simulink model "SHEV_Camaro_PwrLossMdl"  (R2018b)
settings: Solver=ode2  StartTime=0.0  StopTime=simDrv.time_s(end)  FixedStep=t_step  RelTol=1e-3
values from neighbouring files (symbols this model uses):
  A123_ESS =     [PwrLossMdl_A123Battery.mat]
  contMotTrq = [180;180;180;180;180;180;180;180;170]    [startPwrLossMdl.m]
  cs_ll = 0.15    [startPwrLossMdl.m]
  cs_ul = 0.25    [startPwrLossMdl.m]
  E85_LHV = 30000    [startPwrLossMdl.m]
  mot_gbx_rat = 4.2    [startPwrLossMdl.m]
  rho_fuel_gpL = 783    [startPwrLossMdl.m]
  simDrv = EEC_Single    [startPwrLossMdl.m]
  t_step = 0.1    [startPwrLossMdl.m]
  tire_rad_m = 0.346    [startPwrLossMdl.m]
  V_fuel_init_gal = 7    [startPwrLossMdl.m]
undefined symbols (not defined in the file or in its folder): adj_motEffMap, adjbsfc_map, adjbsfc_spdbpt, adjbsfc_trqbpt, C1, C2, DiscIntNeverNeededParam, motSpdVec, motTrqVec, N_OptResults, R0, R1, R2, soc_bpt
libraries: simulink x7, custom_func x1, dspstat3 x1
PauseFcn:
  | runOptSHEV_DP_FwdProp
settings Model: Creator=Aman-Home  LastModifiedBy=amankalia

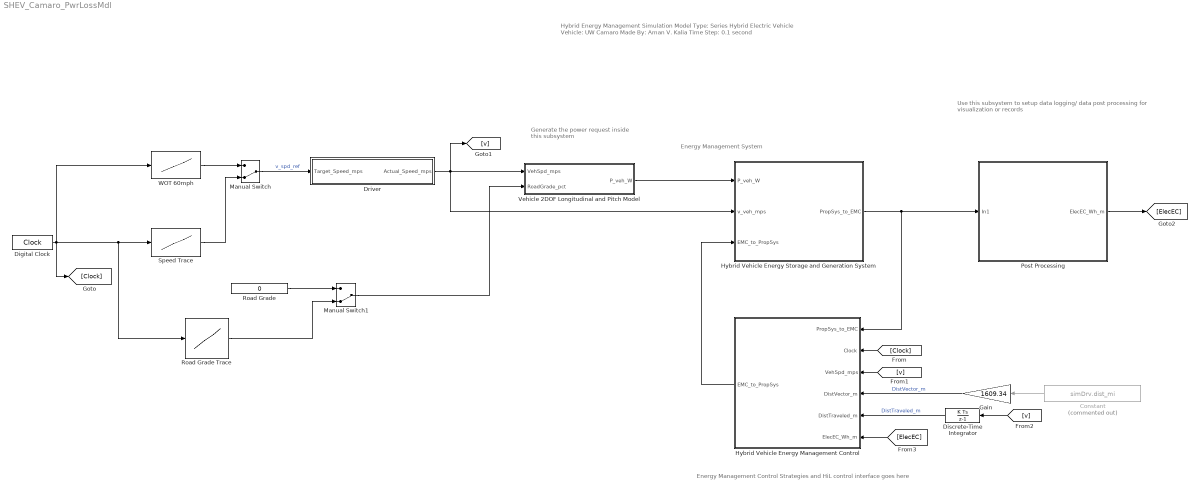
== system SHEV_Camaro_PwrLossMdl ==
  note: Energy Management Control Strategies and HiL control interface goes here
  note: Hybrid Energy Management Simulation Model
      | Type: Series Hybrid Electric Vehicle
      | Vehicle: UW Camaro
      | Made By: Aman V. Kalia
      | Time Step: 0.1 second
  note: Use this subsystem to setup data logging/ data post processing
      | for visualization or records
  note: Generate the power request inside
      | this subsystem
  note: Energy Management System
  Constant : Constant  Commented=on  Value=simDrv.dist_mi
  Digital Clock : DigitalClock  SampleTime=t_step
  Discrete-Time Integrator : DiscreteIntegrator  SampleTime=t_step  ICPrevOutput=DiscIntNeverNeededParam  ICPrevScaledInput=DiscIntNeverNeededParam
  Driver : Subsystem
  Gain : Gain  Gain=1609.34
  Hybrid Vehicle Energy Management Control : Subsystem
  Hybrid Vehicle Energy Storage and Generation System : Subsystem
  Manual Switch : ManualSwitch  CurrentSetting=0
  Manual Switch1 : ManualSwitch  CurrentSetting=0
  Post Processing : Subsystem
  Road Grade : Constant  Value=0
  Road Grade Trace : Lookup_n-D  NumberOfTableDimensions=1  BreakpointsForDimension1=simDrv.time_s  Table=simDrv.grade_pct  ExtrapMethod=Clip  InternalRulePriority=Speed  RndMeth=Simplest  InputSameDT=on
  Speed Trace : Lookup_n-D  NumberOfTableDimensions=1  BreakpointsForDimension1=simDrv.time_s  Table=simDrv.spd_mps  ExtrapMethod=Clip  InternalRulePriority=Speed  RndMeth=Simplest  InputSameDT=on
  Vehicle 2DOF Longitudinal and Pitch Model : Subsystem
  WOT 60mph : Lookup_n-D  NumberOfTableDimensions=1  BreakpointsForDimension1=[0,5,10,simDrv.time_s(end)]  Table=[0,0,60,60] * 0.447  ExtrapMethod=Clip  InternalRulePriority=Speed  RndMeth=Simplest  InputSameDT=on
  wires:
  Manual Switch/1 -> Driver/1(Target_Speed_mps)  "v_spd_ref"
  Driver/1(Actual_Speed_mps) -> [v], Hybrid Vehicle Energy Storage and Generation System/2(v_veh_mps), Vehicle 2DOF Longitudinal and Pitch Model/1(VehSpd_mps)
  Hybrid Vehicle Energy Management Control/1(EMC_to_PropSys) -> Hybrid Vehicle Energy Storage and Generation System/3(EMC_to_PropSys)
  Hybrid Vehicle Energy Storage and Generation System/1(PropSys_to_EMC) -> Hybrid Vehicle Energy Management Control/1(PropSys_to_EMC), Post Processing/1(In1)
  Vehicle 2DOF Longitudinal and Pitch Model/1(P_veh_W) -> Hybrid Vehicle Energy Storage and Generation System/1(P_veh_W)
  Manual Switch1/1 -> Vehicle 2DOF Longitudinal and Pitch Model/2(RoadGrade_pct)
  Digital Clock/1 -> WOT 60mph/1, [Clock], Road Grade Trace/1, Speed Trace/1
  Speed Trace/1 -> Manual Switch/2
  Road Grade/1 -> Manual Switch1/1
  Road Grade Trace/1 -> Manual Switch1/2
  [Clock] -> Hybrid Vehicle Energy Management Control/2(Clock)
  [v] -> Hybrid Vehicle Energy Management Control/3(VehSpd_mps)
  Constant/1 -> Gain/1
  [v] -> Discrete-Time Integrator/1
  Discrete-Time Integrator/1 -> Hybrid Vehicle Energy Management Control/5(DistTraveled_m)  "DistTraveled_m"
  Gain/1 -> Hybrid Vehicle Energy Management Control/4(DistVector_m)  "DistVector_m"
  WOT 60mph/1 -> Manual Switch/1
  Post Processing/1(ElecEC_Wh_m) -> [ElecEC]
  [ElecEC] -> Hybrid Vehicle Energy Management Control/6(ElecEC_Wh_m)

== system SHEV_Camaro_PwrLossMdl/Driver ==
  Target_Speed_mps : Inport
  Actual_Speed_mps : Outport
  wires:
  Target_Speed_mps/1 -> Actual_Speed_mps/1

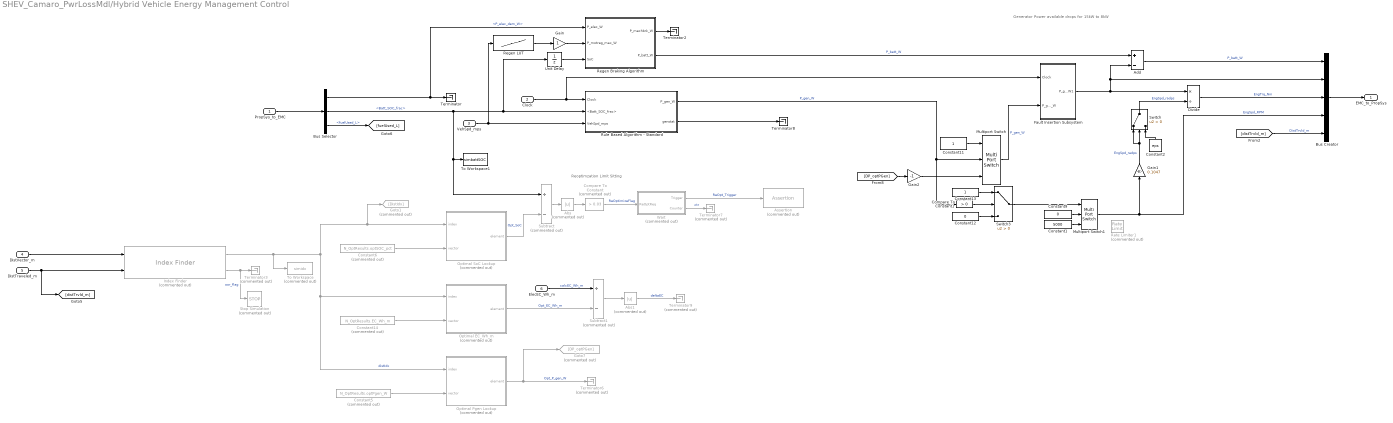
== system SHEV_Camaro_PwrLossMdl/Hybrid Vehicle Energy Management Control ==
  note: Generator Power available drops for 15kW to 8kW
  note: Reoptimzation Limit Sitting
  PropSys_to_EMC : Inport
  Clock : Inport  Port=2
  VehSpd_mps : Inport  Port=3
  DistVector_m : Inport  Port=4
  DistTraveled_m : Inport  Port=5
  ElecEC_Wh_m : Inport  Port=6
  Abs : Abs  Commented=on
  Abs1 : Abs  Commented=on
  Add : Sum  Inputs=+-
  Assertion : Assertion  Commented=on  AssertionFailFcn=set_param(bdroot,'SimulationCommand','pause');  StopWhenAssertionFail=off
  Bus Creator : BusCreator  Inputs=5
  Bus Selector : BusSelector  OutputSignals=P_elec_dem_W,Batt_SOC_frac,fuelUsed_L
  Compare To Constant : simulink/Logic and Bit Operations/Compare To Constant  Commented=on  relop=>  const=0.03  OutDataTypeStr=boolean
  Compare To Constant1 : simulink/Logic and Bit Operations/Compare To Constant  relop=>  const=0  OutDataTypeStr=boolean
  Constant1 : Constant  Value=5000
  Constant11 : Constant
  Constant12 : Constant  Value=0
  Constant13 : Constant
  Constant14 : Constant  Commented=on  Value=N_OptResults.EC_Wh_m
  Constant2 : Constant  Value=eps
  Constant5 : Constant  Commented=on  Value=N_OptResults.optPgen_W
  Constant6 : Constant  Commented=on  Value=N_OptResults.optSOC_pct
  Constant9 : Constant  Value=0
  Divide : Product  Inputs=*/
  Fault Insertion Subsystem : Subsystem  mask{FaultDec=off}
      mask prompts: FaultDec "Insert Fault"
      mask DialogControl DescGroupVar Prompt: Fault Insertion Block
      mask DialogControl DescTextVar Prompt: Select "Insert Fault" to enable fault insertion. Deselect to turn it off.
  Gain : Gain
  Gain1 : Gain  Gain=0.1047
  Gain2 : Gain  Gain=-1
  Goto1 : Goto  Commented=on  GotoTag=DistIdx
  Goto7 : Goto  Commented=on  GotoTag=DP_optPGen
  Index Finder : custom_func/Index Finder  Commented=on  SystemSampleTime=-1
  Multiport Switch : MultiPortSwitch  Inputs=2
  Multiport Switch1 : MultiPortSwitch  DataPortOrder=Zero-based contiguous  Inputs=2  zeroidx=on
  Optimal EC_Wh_m : MATLAB Function  Commented=on  TreatAsAtomicUnit=on
  Optimal Pgen Lookup : MATLAB Function  Commented=on  TreatAsAtomicUnit=on
  Optimal SoC Lookup : MATLAB Function  Commented=on  TreatAsAtomicUnit=on
  Rate Limiter1 : RateLimiter  Commented=on  RisingSlewLimit=75  FallingSlewLimit=-1000  SampleTimeMode=inherited
  Regen Braking Algorithm : Stateflow chart  TreatAsAtomicUnit=on
  Regen LUT : Lookup_n-D  NumberOfTableDimensions=1  BreakpointsForDimension1=[0 2.6 5.2 7.8 10.4 13 15.6 18.2 20.8 23.4 26 28.6 31.2 33.8 38]  Table=[0 0 -1250 -3000 -5500 -8000 -10250 -12500 -13750 -14000 -14500 -15000 -15000 -15000 -15000]  InternalRulePriority=Speed  RndMeth=Simplest  InputSameDT=on
  Rule Based Algorithm - Standard : Subsystem
  Stop Simulation : Stop  Commented=on
  Subtract : Sum  Commented=on  Inputs=+-
  Subtract1 : Sum  Commented=on  Inputs=+-
  Switch : Switch  Criteria=u2 > Threshold
  Switch3 : Switch  Criteria=u2 > Threshold
  Terminator : Terminator
  Terminator2 : Terminator
  Terminator{3,6..7,9} (4 alike) : Terminator  Commented=on
  Terminator8 : Terminator
  To Workspace : ToWorkspace  Commented=on  VariableName=simidx  SaveFormat=Timeseries  SampleTime=1
      settings: Save2DSignal=2-D array (concatenate along first dimension)
  To Workspace1 : ToWorkspace  VariableName=simbattSOC  SaveFormat=Timeseries  SampleTime=1
  Unit Delay : UnitDelay  SampleTime=-1
  Wait : Stateflow chart  Commented=on  TreatAsAtomicUnit=on
  EMC_to_PropSys : Outport
  wires:
  Bus Creator/1 -> EMC_to_PropSys/1
  Add/1 -> Bus Creator/1  "P_batt_W"
  Divide/1 -> Bus Creator/3  "EngTrq_Nm"
  Multiport Switch1/1 -> Gain1/1, Bus Creator/4  "EngSpd_RPM"
  PropSys_to_EMC/1 -> Bus Selector/1
  Bus Selector/1 -> Terminator/1, Regen Braking Algorithm/1(P_elec_W)  "<P_elec_dem_W>"
  Regen LUT/1 -> Gain/1
  Regen Braking Algorithm/1(P_mechbrk_W) -> Terminator2/1
  Gain/1 -> Regen Braking Algorithm/2(P_motreg_max_W)
  Constant9/1 -> Multiport Switch1/2
  Constant1/1 -> Multiport Switch1/3
  Switch/1 -> Divide/2  "EngSpd_radps"
  Gain1/1 -> Switch/1, Switch/2  "EngSpd_radps"
  Constant2/1 -> Switch/3
  Regen Braking Algorithm/2(P_batt_W) -> Add/1  "P_batt_W"
  Clock/1 -> Fault Insertion Subsystem/1(Clock), Rule Based Algorithm - Standard/1(Clock)
  Bus Selector/2 -> To Workspace1/1, Subtract/1, Unit Delay/1, Rule Based Algorithm - Standard/2(<Batt_SOC_frac>)  "<Batt_SOC_frac>"
  VehSpd_mps/1 -> Regen LUT/1, Rule Based Algorithm - Standard/3(VehSpd_mps)
  Switch3/1 -> Multiport Switch1/1
  DistVector_m/1 -> Index Finder/1
  DistTraveled_m/1 -> [distTrvld_m], Index Finder/2
  Index Finder/1 -> To Workspace/1, Goto1/1, Optimal SoC Lookup/1(index), Optimal EC_Wh_m/1(index), Optimal Pgen Lookup/1(index)  "distIdx"
  Index Finder/2 -> Terminator3/1, Stop Simulation/1  "oor_flag"
  Subtract/1 -> Abs/1
  Abs/1 -> Compare To Constant/1
  Compare To Constant/1 -> Wait/1(ReOptReq)  "ReOptimizeFlag"
  Wait/1(Trigger) -> Assertion/1  "ReOpt_Trigger"
  Optimal Pgen Lookup/1(element) -> Goto7/1, Terminator6/1  "Opt_P_gen_W"
  Wait/2(Counter) -> Terminator7/1  "ctr"
  Constant5/1 -> Optimal Pgen Lookup/2(vector)
  Optimal SoC Lookup/1(element) -> Subtract/2  "Opt_SoC"
  Constant6/1 -> Optimal SoC Lookup/2(vector)
  Bus Selector/3 -> [fuelUsed_L]  "<fuelUsed_L>"
  [DP_optPGen] -> Gain2/1
  Gain2/1 -> Multiport Switch/3
  Rule Based Algorithm - Standard/1(P_gen_W) -> Compare To Constant1/1, Multiport Switch/2  "P_gen_W"
  Constant11/1 -> Multiport Switch/1
  Rule Based Algorithm - Standard/2(genstat) -> Terminator8/1
  Compare To Constant1/1 -> Switch3/2
  Constant12/1 -> Switch3/3
  Constant13/1 -> Switch3/1
  [distTrvld_m] -> Bus Creator/5  "DistTrvld_m"
  Constant14/1 -> Optimal EC_Wh_m/2(vector)
  Optimal EC_Wh_m/1(element) -> Subtract1/2  "Opt_EC_Wh_m"
  ElecEC_Wh_m/1 -> Subtract1/1  "calcEC_Wh_m"
  Subtract1/1 -> Abs1/1
  Abs1/1 -> Terminator9/1  "deltaEC"
  Unit Delay/1 -> Regen Braking Algorithm/3(SoC)
  Fault Insertion Subsystem/1(P_gen_W1) -> Add/2, Bus Creator/2, Divide/1
  Multiport Switch/1 -> Fault Insertion Subsystem/2(P_gen_W)  "P_gen_W"

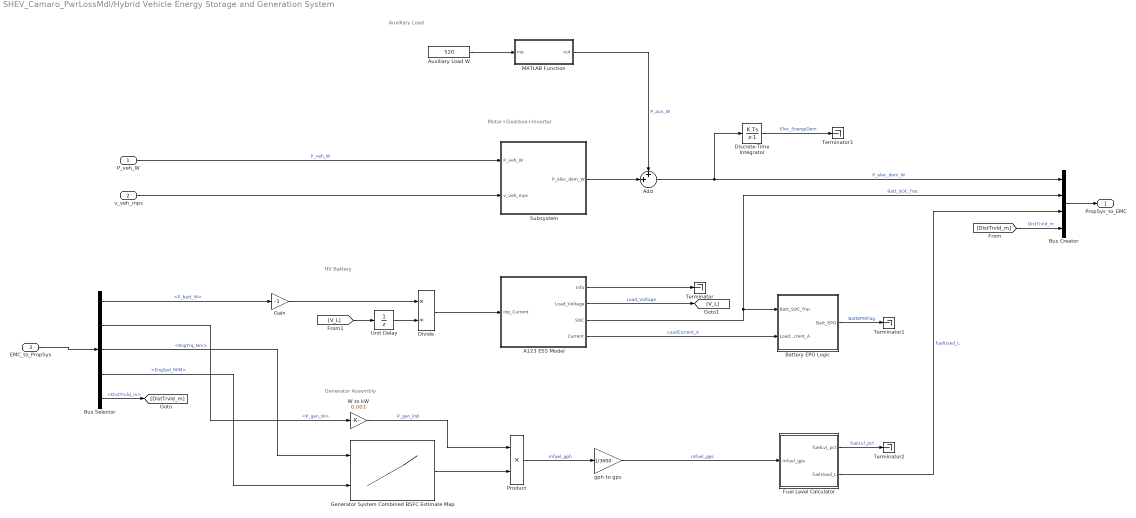
== system SHEV_Camaro_PwrLossMdl/Hybrid Vehicle Energy Storage and Generation System ==
  note: HV Battery
  note: Generator Assembly
  note: Auxiliary Load
  note: Motor+Gearbox+Inverter
  P_veh_W : Inport
  v_veh_mps : Inport  Port=2
  EMC_to_PropSys : Inport  Port=3
  A123 ESS Model : Subsystem  AncestorBlock=lib_ESS/A123 ESS Model  mask{Q_max_cell=A123_ESS.Q_cell_max_Ah, Np=A123_ESS.Np, Ns=A123_ESS.Ns, Nmod=A123_ESS.Nmod, soc_init=A123_ESS.Init_soc, soc_bpt=soc_bpt, R0=R0, R1=R1, C1=C1, R2=R2, C2=C2, t_step=t_step}
      mask prompts: Q_max_cell "Max cell capacity [Ah]:"; Np "Number of cells in parallel []:"; Ns "Numer of cells in series []:"; Nmod "Number of modules []:"; soc_init "Initial SoC/100 []:"; soc_bpt "SoC break points []:"; R0 "Internal resistance vector []:"; R1 "RC1 resistance vector []:"; C1 "RC1 capacitance vector []:"; R2 "RC2 resistance vector []:"; C2 "RC2 capacitance vector []:"; t_step "Simulation time step:"
      mask DialogControl DescGroupVar Prompt: Parameter Settings
      mask DialogControl DescTextVar Prompt: This model emulates an A123 ESS used by UW EcoCAR Team.
      mask DialogControl BatParamGroupVar Prompt: Battery Parameters
      mask DialogControl EstParamGroupVar Prompt: Estimated RC Parameters
      mask DialogControl MiscSettGroupVar Prompt: Miscellaneous Settings
  Add : Sum  Inputs=++|
  Auxiliary Load W : Constant  Value=520
  Battery EPO Logic : Subsystem
  Bus Creator : BusCreator  Inputs=4
  Bus Selector : BusSelector  OutputSignals=P_batt_W,P_gen_W,EngTrq_Nm,EngSpd_RPM,DistTrvld_m
  Discrete-Time Integrator : DiscreteIntegrator  SampleTime=t_step  ICPrevOutput=DiscIntNeverNeededParam  ICPrevScaledInput=DiscIntNeverNeededParam
  Divide : Product  Inputs=*/
  Fuel Level Calculator : Subsystem
  Gain : Gain  Gain=-1
  Generator System Combined BSFC Estimate Map : Lookup_n-D  BreakpointsForDimension1=adjbsfc_trqbpt  BreakpointsForDimension2=adjbsfc_spdbpt  Table=adjbsfc_map  InternalRulePriority=Speed  RndMeth=Simplest  InputSameDT=on
  MATLAB Function : MATLAB Function  TreatAsAtomicUnit=on
  Product : Product
  Subsystem : Subsystem
  Terminator{,1..3} (4 alike) : Terminator
  Unit Delay : UnitDelay  InitialCondition=A123_ESS.Ns * A123_ESS.Nmod * 3.4  SampleTime=-1
  W to kW : Gain  Gain=0.001
  gph to gps : Gain  Gain=1/3600
  PropSys_to_EMC : Outport
  wires:
  P_veh_W/1 -> Subsystem/1(P_veh_W)  "P_veh_W"
  v_veh_mps/1 -> Subsystem/2(v_veh_mps)
  Auxiliary Load W/1 -> MATLAB Function/1(inp)
  Subsystem/1(P_elec_dem_W) -> Add/2
  MATLAB Function/1(out) -> Add/1  "P_aux_W"
  Add/1 -> Discrete-Time Integrator/1, Bus Creator/1  "P_elec_dem_W"
  Divide/1 -> A123 ESS Model/1(Inp_Current)
  A123 ESS Model/2(Load_Voltage) -> [V_L]  "Load_Voltage"
  [V_L] -> Unit Delay/1
  A123 ESS Model/1(Info) -> Terminator/1
  A123 ESS Model/3(SOC) -> Bus Creator/2, Battery EPO Logic/1(Batt_SOC_frac)  "Batt_SOC_frac"
  Bus Selector/3 -> Generator System Combined BSFC Estimate Map/1  "<EngTrq_Nm>"
  Bus Selector/4 -> Generator System Combined BSFC Estimate Map/2  "<EngSpd_RPM>"
  EMC_to_PropSys/1 -> Bus Selector/1
  Bus Selector/1 -> Gain/1  "<P_batt_W>"
  Bus Selector/2 -> W to kW/1  "<P_gen_W>"
  Generator System Combined BSFC Estimate Map/1 -> Product/2
  W to kW/1 -> Product/1  "P_gen_kW"
  Product/1 -> gph to gps/1  "mfuel_gph"
  Bus Creator/1 -> PropSys_to_EMC/1
  Unit Delay/1 -> Divide/2
  Gain/1 -> Divide/1
  A123 ESS Model/4(Current) -> Battery EPO Logic/2(LoadCurrent_A)  "LoadCurrent_A"
  Battery EPO Logic/1(Batt_EPO) -> Terminator1/1  "BattEPOFlag"
  gph to gps/1 -> Fuel Level Calculator/1(mfuel_gps)  "mfuel_gps"
  Fuel Level Calculator/1(fuelLvl_pct) -> Terminator2/1  "fuelLvl_pct"
  Discrete-Time Integrator/1 -> Terminator3/1  "Elec_EnergyDem"
  Fuel Level Calculator/2(fuelUsed_L) -> Bus Creator/3  "fuelUsed_L"
  Bus Selector/5 -> [DistTrvld_m]  "<DistTrvld_m>"
  [DistTrvld_m] -> Bus Creator/4  "DistTrvld_m"

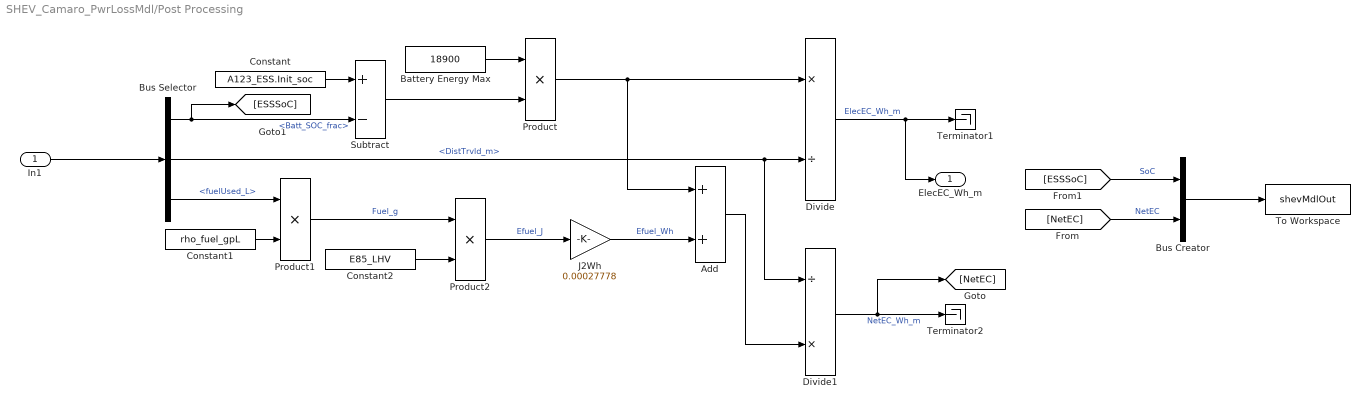
== system SHEV_Camaro_PwrLossMdl/Post Processing ==
  In1 : Inport
  Add : Sum
  Battery Energy Max : Constant  Value=18900
  Bus Creator : BusCreator  Inputs=2
  Bus Selector : BusSelector  OutputSignals=Batt_SOC_frac,DistTrvld_m,fuelUsed_L
  Constant : Constant  Value=A123_ESS.Init_soc
  Constant1 : Constant  Value=rho_fuel_gpL
  Constant2 : Constant  Value=E85_LHV
  Divide : Product  Inputs=*/
  Divide1 : Product  Inputs=/*
  J2Wh : Gain  Gain=0.00027778
  Product : Product
  Product1 : Product
  Product2 : Product
  Subtract : Sum  Inputs=+-
  Terminator1 : Terminator
  Terminator2 : Terminator
  To Workspace : ToWorkspace  VariableName=shevMdlOut  SaveFormat=Timeseries  SampleTime=-1
  ElecEC_Wh_m : Outport
  wires:
  In1/1 -> Bus Selector/1
  Bus Selector/1 -> [ESSSoC], Subtract/2  "<Batt_SOC_frac>"
  Constant/1 -> Subtract/1
  Subtract/1 -> Product/2
  Battery Energy Max/1 -> Product/1
  Product/1 -> Add/1, Divide/1
  Bus Selector/2 -> Divide1/1, Divide/2  "<DistTrvld_m>"
  Bus Selector/3 -> Product1/1  "<fuelUsed_L>"
  Divide/1 -> ElecEC_Wh_m/1, Terminator1/1  "ElecEC_Wh_m"
  Constant1/1 -> Product1/2
  Product1/1 -> Product2/1  "Fuel_g"
  Constant2/1 -> Product2/2
  Product2/1 -> J2Wh/1  "Efuel_J"
  J2Wh/1 -> Add/2  "Efuel_Wh"
  Add/1 -> Divide1/2
  Divide1/1 -> [NetEC], Terminator2/1  "NetEC_Wh_m"
  Bus Creator/1 -> To Workspace/1
  [NetEC] -> Bus Creator/2  "NetEC"
  [ESSSoC] -> Bus Creator/1  "SoC"

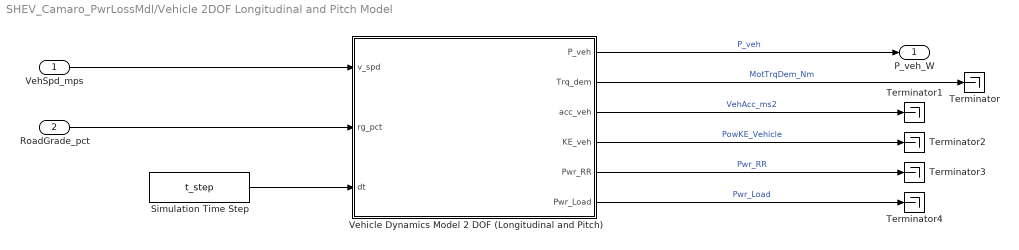
== system SHEV_Camaro_PwrLossMdl/Vehicle 2DOF Longitudinal and Pitch Model ==
  VehSpd_mps : Inport
  RoadGrade_pct : Inport  Port=2
  Simulation Time Step : Constant  Value=t_step
  Terminator{,1..4} (5 alike) : Terminator
  Vehicle Dynamics Model 2 DOF (Longitudinal and Pitch) : MATLAB Function  TreatAsAtomicUnit=on
  P_veh_W : Outport
  wires:
  VehSpd_mps/1 -> Vehicle Dynamics Model 2 DOF (Longitudinal and Pitch)/1(v_spd)
  Vehicle Dynamics Model 2 DOF (Longitudinal and Pitch)/1(P_veh) -> P_veh_W/1  "P_veh"
  RoadGrade_pct/1 -> Vehicle Dynamics Model 2 DOF (Longitudinal and Pitch)/2(rg_pct)
  Simulation Time Step/1 -> Vehicle Dynamics Model 2 DOF (Longitudinal and Pitch)/3(dt)
  Vehicle Dynamics Model 2 DOF (Longitudinal and Pitch)/2(Trq_dem) -> Terminator/1  "MotTrqDem_Nm"
  Vehicle Dynamics Model 2 DOF (Longitudinal and Pitch)/3(acc_veh) -> Terminator1/1  "VehAcc_ms2"
  Vehicle Dynamics Model 2 DOF (Longitudinal and Pitch)/4(KE_veh) -> Terminator2/1  "PowKE_Vehicle"
  Vehicle Dynamics Model 2 DOF (Longitudinal and Pitch)/5(Pwr_RR) -> Terminator3/1  "Pwr_RR"
  Vehicle Dynamics Model 2 DOF (Longitudinal and Pitch)/6(Pwr_Load) -> Terminator4/1  "Pwr_Load"

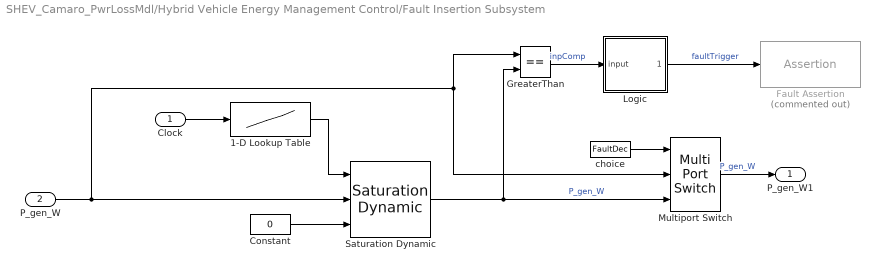
== system SHEV_Camaro_PwrLossMdl/Hybrid Vehicle Energy Management Control/Fault Insertion Subsystem ==
  Clock : Inport
  P_gen_W : Inport  Port=2
  1-D Lookup Table : Lookup_n-D  NumberOfTableDimensions=1  BreakpointsForDimension1=[0,1200,1210,simDrv.time_s(end)]  Table=[15000,15000,8000,8000]  InternalRulePriority=Speed  RndMeth=Simplest  InputSameDT=on
  Constant : Constant  Value=0
  Fault Assertion : Assertion  Commented=on  AssertionFailFcn=|  StopWhenAssertionFail=off
      | set_param(bdroot,'SimulationCommand','pause');
      | disp('## Paused due to fault insertion')
  GreaterThan : RelationalOperator  Operator===  OutDataTypeStr=boolean  RndMeth=Simplest
  Logic : Stateflow chart  TreatAsAtomicUnit=on
  Multiport Switch : MultiPortSwitch  DataPortOrder=Zero-based contiguous  Inputs=2  zeroidx=on
  Saturation Dynamic : simulink/Discontinuities/Saturation Dynamic  OutMin=[]  OutMax=[]  OutDataTypeStr=Inherit: Same as second input  OutDataType=fixdt(1, 16)  OutScaling=2^-10  DoSatur=off
  choice : Constant  Value=FaultDec
  P_gen_W1 : Outport
  wires:
  Multiport Switch/1 -> P_gen_W1/1  "P_gen_W"
  Constant/1 -> Saturation Dynamic/3
  Clock/1 -> 1-D Lookup Table/1
  P_gen_W/1 -> Multiport Switch/2, GreaterThan/1, Saturation Dynamic/2
  1-D Lookup Table/1 -> Saturation Dynamic/1
  Saturation Dynamic/1 -> GreaterThan/2, Multiport Switch/3  "P_gen_W"
  choice/1 -> Multiport Switch/1
  GreaterThan/1 -> Logic/1(input)  "inpComp"
  Logic/1(trigger) -> Fault Assertion/1  "faultTrigger"

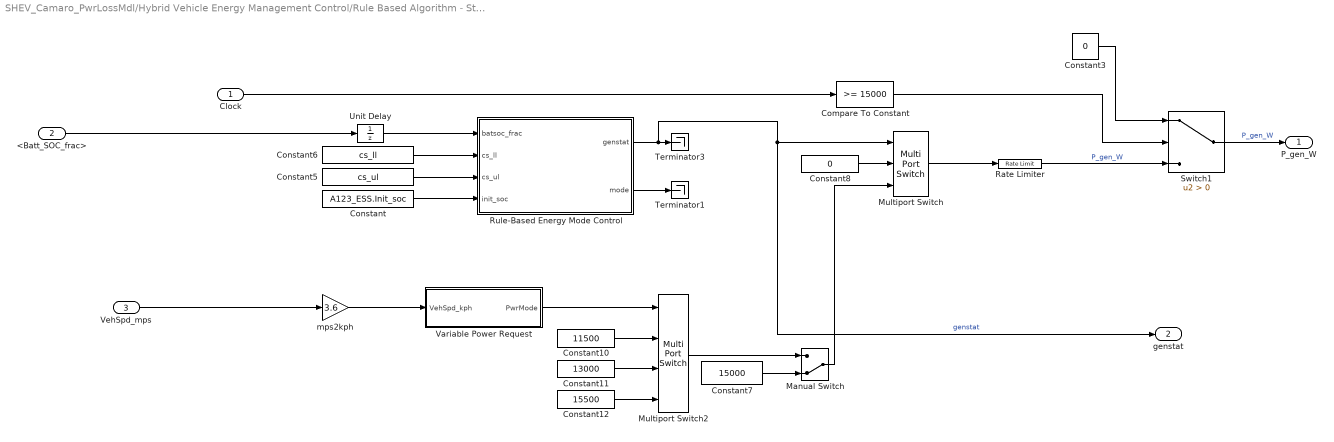
== system SHEV_Camaro_PwrLossMdl/Hybrid Vehicle Energy Management Control/Rule Based Algorithm - Standard ==
  Clock : Inport
  <Batt_SOC_frac> : Inport  Port=2
  VehSpd_mps : Inport  Port=3
  Compare To Constant : simulink/Logic and Bit Operations/Compare To Constant  relop=>=  const=15000  OutDataTypeStr=boolean
  Constant : Constant  Value=A123_ESS.Init_soc
  Constant10 : Constant  Value=11500
  Constant11 : Constant  Value=13000
  Constant12 : Constant  Value=15500
  Constant3 : Constant  Value=0
  Constant5 : Constant  Value=cs_ul
  Constant6 : Constant  Value=cs_ll
  Constant7 : Constant  Value=15000
  Constant8 : Constant  Value=0
  Manual Switch : ManualSwitch  CurrentSetting=0
  Multiport Switch : MultiPortSwitch  DataPortOrder=Zero-based contiguous  Inputs=2  zeroidx=on
  Multiport Switch2 : MultiPortSwitch  DataPortOrder=Zero-based contiguous  zeroidx=on
  Rate Limiter : RateLimiter  RisingSlewLimit=250  FallingSlewLimit=-4500  SampleTimeMode=inherited
  Rule-Based Energy Mode Control : Stateflow chart  TreatAsAtomicUnit=on
  Switch1 : Switch  Criteria=u2 > Threshold
  Terminator1 : Terminator
  Terminator3 : Terminator
  Unit Delay : UnitDelay  SampleTime=-1
  Variable Power Request : MATLAB Function  TreatAsAtomicUnit=on
  mps2kph : Gain  Gain=3.6
  P_gen_W : Outport
  genstat : Outport  Port=2
  wires:
  Multiport Switch2/1 -> Manual Switch/1
  Constant12/1 -> Multiport Switch2/4
  Constant11/1 -> Multiport Switch2/3
  Variable Power Request/1(PwrMode) -> Multiport Switch2/1
  Constant3/1 -> Switch1/1
  <Batt_SOC_frac>/1 -> Unit Delay/1
  Constant/1 -> Rule-Based Energy Mode Control/4(init_soc)
  Constant10/1 -> Multiport Switch2/2
  Constant8/1 -> Multiport Switch/2
  Clock/1 -> Compare To Constant/1
  Multiport Switch/1 -> Rate Limiter/1
  Rule-Based Energy Mode Control/2(mode) -> Terminator1/1
  Constant7/1 -> Manual Switch/2
  Rule-Based Energy Mode Control/1(genstat) -> genstat/1, Multiport Switch/1, Terminator3/1  "genstat"
  VehSpd_mps/1 -> mps2kph/1
  Unit Delay/1 -> Rule-Based Energy Mode Control/1(batsoc_frac)
  mps2kph/1 -> Variable Power Request/1(VehSpd_kph)
  Constant5/1 -> Rule-Based Energy Mode Control/3(cs_ul)
  Compare To Constant/1 -> Switch1/2
  Rate Limiter/1 -> Switch1/3  "P_gen_W"
  Constant6/1 -> Rule-Based Energy Mode Control/2(cs_ll)
  Manual Switch/1 -> Multiport Switch/3
  Switch1/1 -> P_gen_W/1  "P_gen_W"

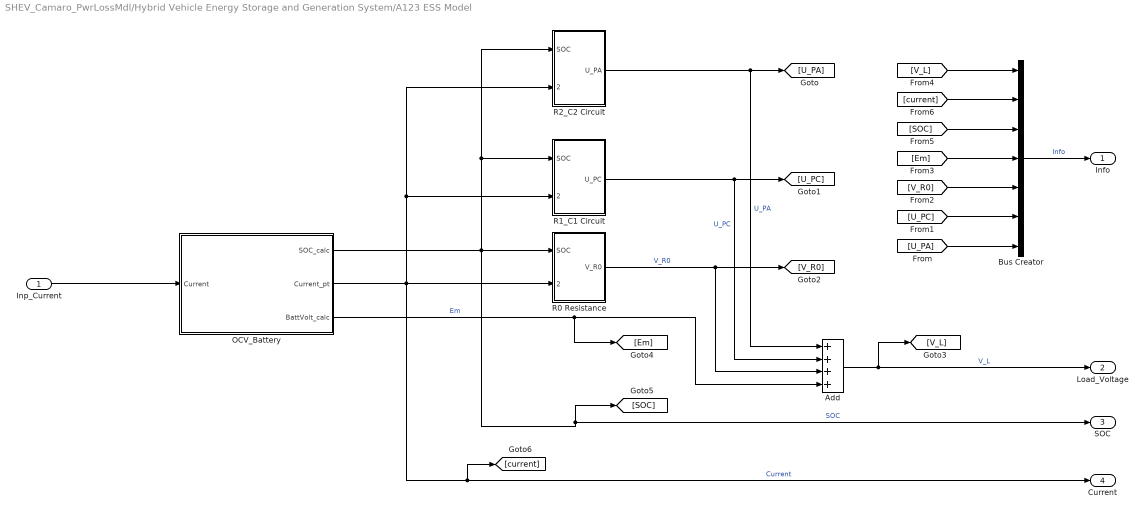
== system SHEV_Camaro_PwrLossMdl/Hybrid Vehicle Energy Storage and Generation System/A123 ESS Model ==
  Inp_Current : Inport
  Add : Sum  Inputs=++++
  Bus Creator : BusCreator  Inputs=7
  OCV_Battery : Subsystem
  R0 Resistance : Subsystem
  R1_C1 Circuit : Subsystem
  R2_C2 Circuit : Subsystem
  Info : Outport
  Load_Voltage : Outport  Port=2
  SOC : Outport  Port=3
  Current : Outport  Port=4
  wires:
  [SOC] -> Bus Creator/3
  [U_PA] -> Bus Creator/7
  Inp_Current/1 -> OCV_Battery/1(Current)
  [current] -> Bus Creator/2
  Add/1 -> Load_Voltage/1, [V_L]  "V_L"
  [Em] -> Bus Creator/4
  R0 Resistance/1(V_R0) -> [V_R0], Add/3  "V_R0"
  R2_C2 Circuit/1(U_PA) -> Add/1, [U_PA]  "U_PA"
  OCV_Battery/2(Current_pt) -> Current/1, [current], R2_C2 Circuit/2(Current), R1_C1 Circuit/2(Current), R0 Resistance/2(Current)  "Current"
  OCV_Battery/1(SOC_calc) -> SOC/1, [SOC], R2_C2 Circuit/1(SOC), R1_C1 Circuit/1(SOC), R0 Resistance/1(SOC)  "SOC"
  R1_C1 Circuit/1(U_PC) -> Add/2, [U_PC]  "U_PC"
  [U_PC] -> Bus Creator/6
  OCV_Battery/3(BattVolt_calc) -> [Em], Add/4  "Em"
  [V_R0] -> Bus Creator/5
  Bus Creator/1 -> Info/1  "Info"
  [V_L] -> Bus Creator/1

== system SHEV_Camaro_PwrLossMdl/Hybrid Vehicle Energy Storage and Generation System/Battery EPO Logic ==
  note: Discharge Current is negative
  Batt_SOC_frac : Inport
  LoadCurrent_A : Inport  Port=2
  10-second average : dspstat3/Moving Average  Method=Sliding window  ForgettingFactorPort=off  SpecifyWindowLength=on  WindowLength=1000  ForgettingFactor=0.9  SimulateUsing=Code generation
  10sec Discharge Limit Table A123 : Lookup_n-D  BreakpointsForDimension1=A123_ESS.cellTempbpt_C  BreakpointsForDimension2=A123_ESS.socbpt  Table=A123_ESS.DchgCurrLim_10sAvg_A  InternalRulePriority=Speed  RndMeth=Simplest  InputSameDT=on
  Battery EPO Constraint Logic : Stateflow chart  TreatAsAtomicUnit=on
  CellTemp degC : Constant  Value=35
  Gain1 : Gain  Gain=-1
  Batt_EPO : Outport
  wires:
  Batt_SOC_frac/1 -> 10sec Discharge Limit Table A123/2
  LoadCurrent_A/1 -> 10-second average/1
  Battery EPO Constraint Logic/1(epo_flag) -> Batt_EPO/1  "Batt_EPO"
  10-second average/1 -> Battery EPO Constraint Logic/2(LoadCurr)  "LoadCurrent_10sAvg_A"
  CellTemp degC/1 -> 10sec Discharge Limit Table A123/1
  Gain1/1 -> Battery EPO Constraint Logic/1(DchgCurrLim)
  10sec Discharge Limit Table A123/1 -> Gain1/1

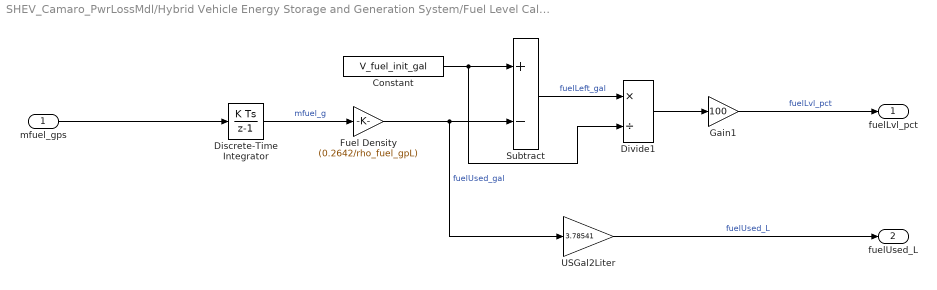
== system SHEV_Camaro_PwrLossMdl/Hybrid Vehicle Energy Storage and Generation System/Fuel Level Calculator ==
  mfuel_gps : Inport
  Constant : Constant  Value=V_fuel_init_gal
  Discrete-Time Integrator : DiscreteIntegrator  SampleTime=-1  ICPrevOutput=DiscIntNeverNeededParam  ICPrevScaledInput=DiscIntNeverNeededParam
  Divide1 : Product  Inputs=*/
  Fuel Density : Gain  Gain=(0.2642/rho_fuel_gpL)
  Gain1 : Gain  Gain=100
  Subtract : Sum  Inputs=+-
  USGal2Liter : Gain  Gain=3.78541
  fuelLvl_pct : Outport
  fuelUsed_L : Outport  Port=2
  wires:
  Divide1/1 -> Gain1/1
  Subtract/1 -> Divide1/1  "fuelLeft_gal"
  Fuel Density/1 -> USGal2Liter/1, Subtract/2  "fuelUsed_gal"
  Constant/1 -> Divide1/2, Subtract/1
  Discrete-Time Integrator/1 -> Fuel Density/1  "mfuel_g"
  mfuel_gps/1 -> Discrete-Time Integrator/1
  Gain1/1 -> fuelLvl_pct/1  "fuelLvl_pct"
  USGal2Liter/1 -> fuelUsed_L/1  "fuelUsed_L"

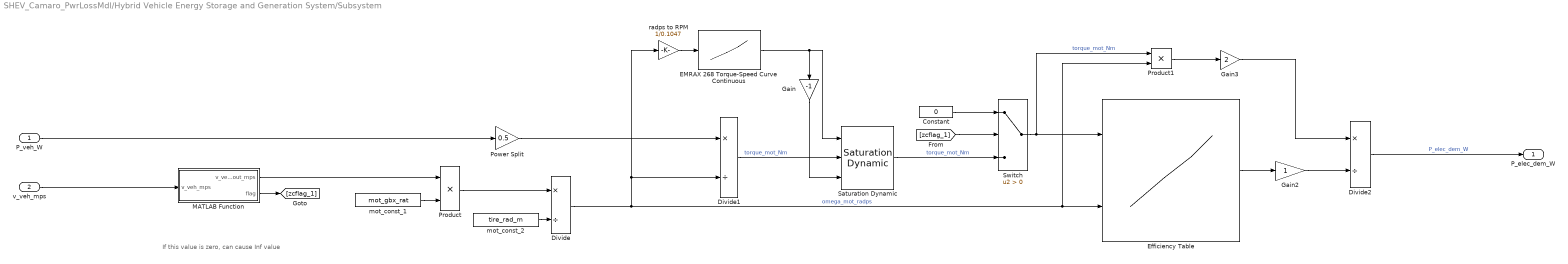
== system SHEV_Camaro_PwrLossMdl/Hybrid Vehicle Energy Storage and Generation System/Subsystem ==
  note: If this value is zero, can cause Inf value
  P_veh_W : Inport
  v_veh_mps : Inport  Port=2
  Constant : Constant  Value=0
  Divide : Product  Inputs=*/
  Divide1 : Product  Inputs=*/
  Divide2 : Product  Inputs=*/
  EMRAX 268 Torque-Speed Curve Continuous : Lookup_n-D  NumberOfTableDimensions=1  BreakpointsForDimension1=motSpdVec  Table=contMotTrq  InternalRulePriority=Speed  RndMeth=Simplest  InputSameDT=on
  Efficiency Table : Lookup_n-D  BreakpointsForDimension1=motTrqVec  BreakpointsForDimension2=motSpdVec  Table=adj_motEffMap  ExtrapMethod=Clip  UseLastTableValue=on  InternalRulePriority=Speed  RndMeth=Simplest  InputSameDT=on
  Gain : Gain  Gain=-1
  Gain2 : Gain
  Gain3 : Gain  Gain=2
  MATLAB Function : MATLAB Function  TreatAsAtomicUnit=on
  Power Split : Gain  Gain=0.5
  Product : Product
  Product1 : Product
  Saturation Dynamic : simulink/Discontinuities/Saturation Dynamic  OutMin=[]  OutMax=[]  OutDataTypeStr=Inherit: Same as second input  OutDataType=fixdt(1, 16)  OutScaling=2^-10  DoSatur=off
  Switch : Switch  Criteria=u2 > Threshold
  mot_const_1 : Constant  Value=mot_gbx_rat
  mot_const_2 : Constant  Value=tire_rad_m
  radps to RPM : Gain  Gain=1/0.1047
  P_elec_dem_W : Outport
  wires:
  Saturation Dynamic/1 -> Switch/3  "torque_mot_Nm"
  [zcflag_1] -> Switch/2
  Switch/1 -> Product1/1, Efficiency Table/1  "torque_mot_Nm"
  Product/1 -> Divide/1
  radps to RPM/1 -> EMRAX 268 Torque-Speed Curve Continuous/1
  Constant/1 -> Switch/1
  MATLAB Function/1(v_veh_out_mps) -> Product/1
  Gain/1 -> Saturation Dynamic/3
  mot_const_1/1 -> Product/2
  EMRAX 268 Torque-Speed Curve Continuous/1 -> Gain/1, Saturation Dynamic/1
  Power Split/1 -> Divide1/1
  v_veh_mps/1 -> MATLAB Function/1(v_veh_mps)
  P_veh_W/1 -> Power Split/1
  Efficiency Table/1 -> Gain2/1
  Divide1/1 -> Saturation Dynamic/2  "torque_mot_Nm"
  mot_const_2/1 -> Divide/2
  Divide/1 -> Divide1/2, radps to RPM/1, Product1/2, Efficiency Table/2  "omega_mot_radps"
  MATLAB Function/2(flag) -> [zcflag_1]
  Product1/1 -> Gain3/1
  Divide2/1 -> P_elec_dem_W/1  "P_elec_dem_W"
  Gain2/1 -> Divide2/2
  Gain3/1 -> Divide2/1

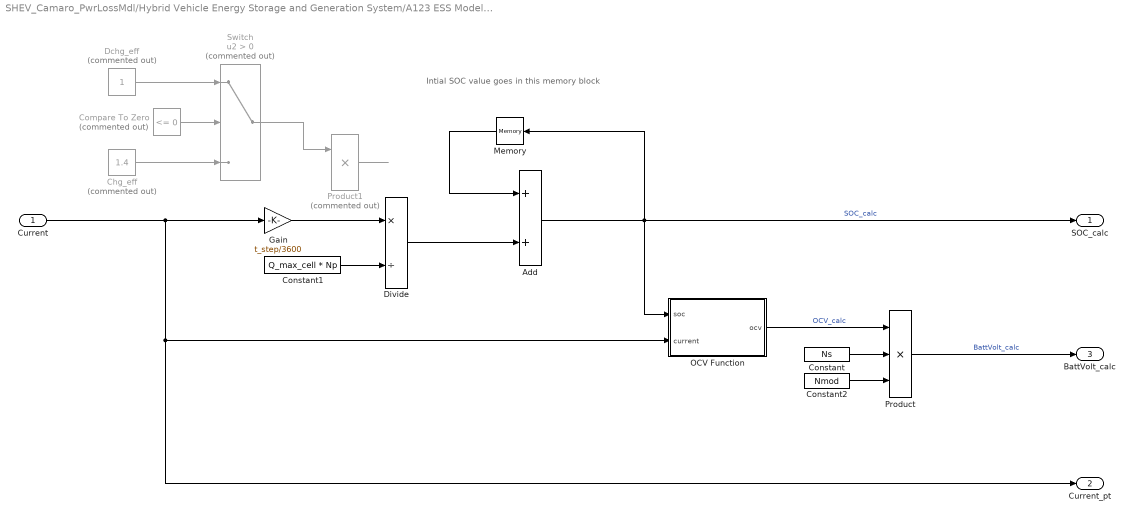
== system SHEV_Camaro_PwrLossMdl/Hybrid Vehicle Energy Storage and Generation System/A123 ESS Model/OCV_Battery ==
  note: Intial SOC value goes in this memory block
  Current : Inport
  Add : Sum
  Chg_eff : Constant  Commented=on  Value=1.4
  Compare To Zero : simulink/Logic and Bit Operations/Compare To Zero  Commented=on  relop=<=  OutDataTypeStr=boolean
  Constant : Constant  Value=Ns
  Constant1 : Constant  Value=Q_max_cell * Np
  Constant2 : Constant  Value=Nmod
  Dchg_eff : Constant  Commented=on
  Divide : Product  Inputs=*/
  Gain : Gain  Gain=t_step/3600
  Memory : Memory  InitialCondition=soc_init  InheritSampleTime=on  LinearizeAsDelay=on
  OCV Function : MATLAB Function  TreatAsAtomicUnit=on
  Product : Product  Inputs=3
  Product1 : Product  Commented=on
  Switch : Switch  Commented=on  Criteria=u2 > Threshold
  SOC_calc : Outport
  Current_pt : Outport  Port=2
  BattVolt_calc : Outport  Port=3
  wires:
  Current/1 -> OCV Function/2(current), Current_pt/1, Gain/1
  Gain/1 -> Divide/1
  Memory/1 -> Add/1
  Constant2/1 -> Product/3
  OCV Function/1(ocv) -> Product/1  "OCV_calc"
  Constant1/1 -> Divide/2
  Add/1 -> SOC_calc/1, OCV Function/1(soc), Memory/1  "SOC_calc"
  Constant/1 -> Product/2
  Divide/1 -> Add/2
  Product/1 -> BattVolt_calc/1  "BattVolt_calc"
  Compare To Zero/1 -> Switch/2
  Dchg_eff/1 -> Switch/1
  Chg_eff/1 -> Switch/3
  Switch/1 -> Product1/1
  Product1/1 -> ?

== system SHEV_Camaro_PwrLossMdl/Hybrid Vehicle Energy Storage and Generation System/A123 ESS Model/R0 Resistance ==
  SOC : Inport
  Current : Inport  Port=2
  Compare To Zero : simulink/Logic and Bit Operations/Compare To Zero  relop=>  OutDataTypeStr=boolean
  Product : Product
  R0 LUT Chg : Lookup_n-D  NumberOfTableDimensions=1  BreakpointsForDimension1=soc_bpt  Table=R0 * 0.05  InternalRulePriority=Speed  RndMeth=Simplest  InputSameDT=on
  R0 LUT Dchg : Lookup_n-D  NumberOfTableDimensions=1  BreakpointsForDimension1=soc_bpt  Table=R0*0.25  InternalRulePriority=Speed  RndMeth=Simplest  InputSameDT=on
  Switch : Switch  Criteria=u2 > Threshold
  V_R0 : Outport
  wires:
  R0 LUT Chg/1 -> Switch/1  "R0"
  SOC/1 -> R0 LUT Chg/1, R0 LUT Dchg/1
  Current/1 -> Compare To Zero/1, Product/2
  Product/1 -> V_R0/1
  Switch/1 -> Product/1
  Compare To Zero/1 -> Switch/2
  R0 LUT Dchg/1 -> Switch/3  "R0"

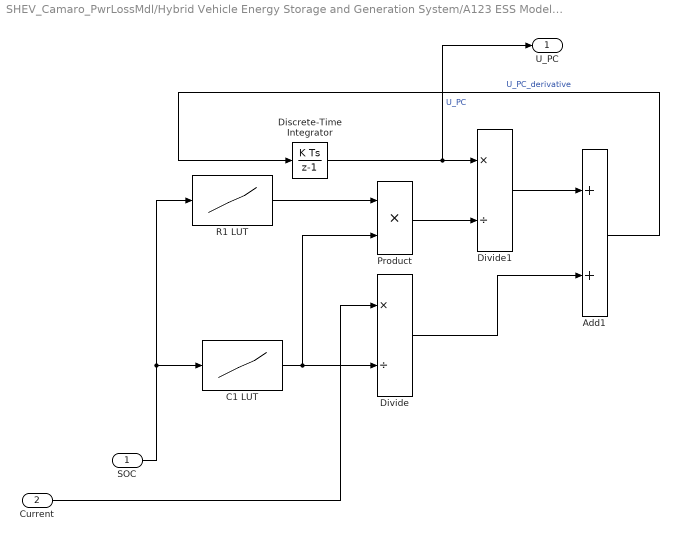
== system SHEV_Camaro_PwrLossMdl/Hybrid Vehicle Energy Storage and Generation System/A123 ESS Model/R1_C1 Circuit ==
  SOC : Inport
  Current : Inport  Port=2
  Add1 : Sum
  C1 LUT : Lookup_n-D  NumberOfTableDimensions=1  BreakpointsForDimension1=soc_bpt  Table=C1  InternalRulePriority=Speed  RndMeth=Simplest  InputSameDT=on
  Discrete-Time Integrator : DiscreteIntegrator  SampleTime=-1  ICPrevOutput=DiscIntNeverNeededParam  ICPrevScaledInput=DiscIntNeverNeededParam
  Divide : Product  Inputs=*/
  Divide1 : Product  Inputs=*/
  Product : Product
  R1 LUT : Lookup_n-D  NumberOfTableDimensions=1  BreakpointsForDimension1=soc_bpt  Table=R1  InternalRulePriority=Speed  RndMeth=Simplest  InputSameDT=on
  U_PC : Outport
  wires:
  Product/1 -> Divide1/2
  SOC/1 -> R1 LUT/1, C1 LUT/1
  Divide1/1 -> Add1/1
  C1 LUT/1 -> Product/2, Divide/2
  Divide/1 -> Add1/2
  R1 LUT/1 -> Product/1
  Discrete-Time Integrator/1 -> U_PC/1, Divide1/1  "U_PC"
  Add1/1 -> Discrete-Time Integrator/1  "U_PC_derivative"
  Current/1 -> Divide/1

== system SHEV_Camaro_PwrLossMdl/Hybrid Vehicle Energy Storage and Generation System/A123 ESS Model/R2_C2 Circuit ==
  SOC : Inport
  Current : Inport  Port=2
  Add1 : Sum
  C2 LUT : Lookup_n-D  NumberOfTableDimensions=1  BreakpointsForDimension1=soc_bpt  Table=C2  InternalRulePriority=Speed  RndMeth=Simplest  InputSameDT=on
  Discrete-Time Integrator : DiscreteIntegrator  SampleTime=-1  ICPrevOutput=DiscIntNeverNeededParam  ICPrevScaledInput=DiscIntNeverNeededParam
  Divide : Product  Inputs=*/
  Divide1 : Product  Inputs=*/
  Product : Product
  R2 LUT : Lookup_n-D  NumberOfTableDimensions=1  BreakpointsForDimension1=soc_bpt  Table=R2  InternalRulePriority=Speed  RndMeth=Simplest  InputSameDT=on
  U_PA : Outport
  wires:
  Product/1 -> Divide1/2
  SOC/1 -> R2 LUT/1, C2 LUT/1
  Divide1/1 -> Add1/1
  C2 LUT/1 -> Product/2, Divide/2
  Divide/1 -> Add1/2
  R2 LUT/1 -> Product/1
  Discrete-Time Integrator/1 -> U_PA/1, Divide1/1  "U_PA"
  Add1/1 -> Discrete-Time Integrator/1  "U_PA_derivative"
  Current/1 -> Divide/1

== matlab function SHEV_Camaro_PwrLossMdl/Hybrid Vehicle Energy Storage and Generation System/Subsystem/MATLAB Function ==
  data: v_veh_mps input; v_veh_out_mps output; flag output
function [v_veh_out_mps,flag] = zerocheck(v_veh_mps)
    % Checks if the input speed is zero. 
    % If zero: sets the flag = 1, to change torque value to zero.
    % If not zero: sets the flag = 0, no change to the the torque value.
    
    if v_veh_mps == 0
        flag = 1;
        v_veh_out_mps = v_veh_mps;
    else
        flag = 0;
        v_veh_out_mps = v_veh_mps;
    end
end

== matlab function SHEV_Camaro_PwrLossMdl/Hybrid Vehicle Energy Storage and Generation System/MATLAB Function ==
  data: inp input; out output
function out = addnoise(inp)
snr = 25;

out = awgn(inp,snr,'measured');

== matlab function SHEV_Camaro_PwrLossMdl/Vehicle 2DOF Longitudinal and Pitch Model/Vehicle Dynamics Model 2 DOF (Longitudinal and Pitch) ==
  data: v_spd input; P_veh output; rg_pct input; dt input; Trq_dem output; acc_veh output; KE_veh output; Pwr_RR output; Pwr_Load output
function [P_veh, Trq_dem, acc_veh, KE_veh, Pwr_RR, Pwr_Load] = vehdyn2dof(v_spd,rg_pct,dt)
    % DESCRIPTION: The 2DOF Longitudinal and Pitch Model for the vehicle
    % uses the longitudinal road load equation comprising of Aerodynamic
    % Resistance, Climbing Resistance, Rolling Resistance as resistive
    % forces on the vehicle.
    %
    % F_veh [N] = F_trac + F_ar + F_cr + F_rr;  --------- (1)
    % P_veh [W] = F_veh [N] * v_veh [m/s];      --------- (2)
    %
    % Note: Pitch dynamics will be added to the model once COG height for
    % the car is determined. Currently only 1DOF longitudinal dynamics
    % exist.
    
    %% Pre-processing
    persistent v_spd_old
    if isempty(v_spd_old)
        v_spd_old = v_spd;
        flag = 1;
    else
        flag = 0;
    end
    alpha = atan(rg_pct/100);
    
    %% Static Parameters
    % -- Vehicle
    A_veh = 0.4;        % [m^2]
    C_d = 0.34;         % drag coefficient [-]
    m_veh = 2012;       %1875;       % [kg]
    P_tire = 32;        % [psi]
    R_tire = 0.346;     % [m]
    N_drvnWhl = 2;      % [-]
    Rat_gbx = 4.2;
    
    % -- Environment
    g = 9.81;           % acceleration due to gravity [m/s^2]
    rho_air = 1.225;    % STP density [kg/m^3]
    
    %% Dynamic Parameters
    C_rr = 0.005 + ((0.06895/P_tire) * ...
        (0.01 + (0.0095 * ((2.778 * (10^-3) * v_spd)^2))));            
    % function of tire pressure and vehicle speed [psi, mps]
    
    %% Vehicle Power Calculation
    if flag == 1
        P_veh = 0;
        Trq_dem = 0; 
        acc_veh = 0;
        KE_veh = 0;
        Pwr_RR = 0;
        Pwr_Load = 0;
    else
        acc_veh = (v_spd - v_spd_old)/dt;
        P_veh = ((m_veh * acc_veh) + ...
            (0.5 * rho_air * A_veh * C_d * (v_spd ^ 2)) + ...
            (m_veh * g * sin(alpha)) + ...
            (C_rr * m_veh * g)) * (v_spd);
        Trq_dem = ((P_veh/v_spd) * R_tire)/((N_drvnWhl * Rat_gbx));
        KE_veh = 0.5 * m_veh * ((v_spd^2) - (v_spd_old^2));
        v_spd_old = v_spd;
        Pwr_RR = (C_rr * m_veh * g) * (v_spd);
        Pwr_Load = ((0.5 * rho_air * A_veh * C_d * (v_spd ^ 2)) + ...
            (m_veh * g * sin(alpha)) + ...
            (C_rr * m_veh * g)) * (v_spd);
    end
    
end

== stateflow chart SHEV_Camaro_PwrLossMdl/Hybrid Vehicle Energy Management Control/Regen Braking Algorithm ==
  note: %P_reg_W
  state NoBraking
    du:
    P_reg_W = 0;
    P_mechbrk_W = 0;
    P_batt_W = P_elec_W;
  state Braking
    state RegenDisabled
      du:
      P_reg_W = 0;
      P_mechbrk_W = P_elec_W;
      P_batt_W = 0;
    state RegenEnabled
      state LightBraking
        du:
        P_reg_W = P_elec_W;
        P_mechbrk_W = P_elec_W - P_reg_W;
        P_batt_W = P_reg_W;
      state HeavyBraking
        du:
        P_reg_W = P_motreg_max_W;
        P_mechbrk_W = P_elec_W - P_reg_W;
        P_batt_W = P_reg_W;
      (default) -> LightBraking
      LightBraking -> HeavyBraking : [P_elec_W <= ...
          | P_motreg_max_W]
      HeavyBraking -> LightBraking : [P_elec_W >= ...
          | P_motreg_max_W]
    (default) -> RegenDisabled
    RegenDisabled -> RegenEnabled : [SoC <= 0.95]
    RegenEnabled -> RegenDisabled : [SoC > 0.95]
  (default) -> NoBraking
  NoBraking -> Braking : [P_elec_W < 0]
  Braking -> NoBraking : [P_elec_W >= 0]
  data: P_elec_W input; P_motreg_max_W input; P_mechbrk_W output double; P_batt_W output double; P_reg_W local double; SoC input

== stateflow chart SHEV_Camaro_PwrLossMdl/Hybrid Vehicle Energy Storage and Generation System/Battery EPO Logic/Battery EPO Constraint Logic ==
  state NoEPO
    du:
    epo_flag = 0;
  state EPO
    du:
    epo_flag = 1;
  (default) -> NoEPO
  NoEPO -> EPO : [LoadCurr < DchgCurrLim]
  EPO -> NoEPO : [LoadCurr >= DchgCurrLim]
  data: DchgCurrLim input; LoadCurr input; epo_flag output double

== stateflow chart SHEV_Camaro_PwrLossMdl/Hybrid Vehicle Energy Management Control/Rule Based Algorithm - Standard/Rule-Based Energy Mode Control ==
  state Initialization
  state CDMode
    du:
    mode = 0;
    genstat = 0;
  state CSModeGen
    du:
    mode = 1;
    genstat = 1;
  state CSModeNoGen
    du:
    mode = 1;
    genstat = 0;
  (default) -> Initialization
  Initialization -> (junction 7) [order 1] : [batsoc_frac <= init_soc && ...
      | batsoc_frac >= cs_ll]
  Initialization -> (junction 10) [order 2] : [batsoc_frac < cs_ll]
  (junction 7) -> CDMode
  (junction 10) -> CSModeGen
  CDMode -> CSModeGen : [batsoc_frac < cs_ll]
  CSModeGen -> CSModeNoGen : [batsoc_frac >= cs_ul]
  CSModeNoGen -> CSModeGen : [batsoc_frac < cs_ll]
  data: batsoc_frac input; cs_ll input; cs_ul input; init_soc input; genstat output double; mode output double

== matlab function SHEV_Camaro_PwrLossMdl/Hybrid Vehicle Energy Management Control/Rule Based Algorithm - Standard/Variable Power Request ==
  data: VehSpd_kph input; PwrMode output
function PwrMode = VarPwrReq(VehSpd_kph)
    if VehSpd_kph >= 0 && VehSpd_kph < 48
        PwrMode = 0;
    elseif VehSpd_kph >= 48 && VehSpd_kph < 97
        PwrMode = 1;
    else
        PwrMode = 2;
    end
end

== matlab function SHEV_Camaro_PwrLossMdl/Hybrid Vehicle Energy Storage and Generation System/A123 ESS Model/OCV_Battery/OCV Function ==
  data: soc input; ocv output; current input
function ocv = fcn(soc, current)

if current < 0
    %% 0-20 Model Fit
    if (soc <= 0.2)
        ocv = 3.17*exp(0.1*soc) - 2.76*exp(-65.25*soc);
    %% 20-80 Model Fit
    elseif (soc > 0.2 && soc <= 0.8)
        ocv = 0.155*soc + 3.2;
        % ocv = 0.165*soc + 3.20; OG
    %% 80-100 Model Fit
    else
        ocv = 0.2*(soc^74.2) + 3.33;
    end
else
    %% 0-20 Model Fit
    if (soc <= 0.2)
        ocv = 3.19*exp(0.098*soc) - 1.09*exp(-48.81*soc);
    %% 20-80 Model Fit
    elseif (soc > 0.2 && soc <= 0.8)
        ocv = 0.148*soc + 3.2;
        % ocv = 0.148*soc + 3.222;
    %% 80-100 Model Fit
    else
        ocv = 0.336*(soc^108.2) + 3.34;
    end
end

== stateflow chart SHEV_Camaro_PwrLossMdl/Hybrid Vehicle Energy Management Control/Wait ==
  state Initialization
    en:
    Counter = 0;
    Trigger = 1;
  state InState
    du:
    Trigger = 1;
  state Wait1
  state Wait
  state OutState
    en:
    Trigger = 0;
    du:
    Trigger = 1;
    ex:
    Trigger = 1;
  (default) -> Initialization
  Initialization -> InState
  Wait1 -> InState : after(5.0,sec)
  Wait -> InState [order 1] : [ReOptReq == 0]
  InState -> Wait : [ReOptReq == 1]
  OutState -> Wait1 : [ReOptReq == 0]
  Wait -> OutState [order 2] : after(5.0,sec){Counter = Counter + 1;}
  data: ReOptReq input; Trigger output double; Counter output double

== stateflow chart SHEV_Camaro_PwrLossMdl/Hybrid Vehicle Energy Management Control/Fault Insertion Subsystem/Logic ==
  state NoFault
    en:
    trigger = 1;
    du:
    trigger = 1;
  state Fault
    en:
    trigger = 0;
    du:
    trigger = 1;
  (default) -> NoFault
  NoFault -> Fault : [input == 0]
  data: input input; trigger output double

== matlab function SHEV_Camaro_PwrLossMdl/Hybrid Vehicle Energy Management Control/Optimal Pgen Lookup ==
  data: index input; element output; vector input
function element = idxLookup(index,vector)
% idxLookup is a custom function that returns element corresponding to
% index in a 1-D vector.
element = vector(index);
end

== matlab function SHEV_Camaro_PwrLossMdl/Hybrid Vehicle Energy Management Control/Optimal SoC Lookup ==
  data: index input; element output; vector input
function element = idxLookup(index,vector)
% idxLookup is a custom function that returns element corresponding to
% index in a 1-D vector.
element = vector(index);
end

== matlab function SHEV_Camaro_PwrLossMdl/Hybrid Vehicle Energy Management Control/Optimal EC_Wh_m ==
  data: index input; element output; vector input
function element = idxLookup(index,vector)
% idxLookup is a custom function that returns element corresponding to
% index in a 1-D vector.
element = vector(index);
end
